simulink subsystem "PMSM_Motor_sref"  (R2025b)
settings: Solver=VariableStepAuto
values from neighbouring files (symbols this model uses):
  B = 1.050e-3    (= 0.00105)    [params_ACT_57BLF02.m]
  J = 1.40e-4    (= 0.00014)    [params_ACT_57BLF02.m]
  Kw = 3.255e-6    (= 3.255e-06)    [params_ACT_57BLF02.m]
  Ld = Ls    (= 0.00019)    [params_ACT_57BLF02.m]
  Lq = Ls    (= 0.00019)    [params_ACT_57BLF02.m]
  p = 4    [params_ACT_57BLF02.m]
  psi = 9.2386e-3    (= 0.0092386)    [params_ACT_57BLF02.m]
  Rs = 0.251    [params_ACT_57BLF02.m]
  T0 = 1.13e-2    (= 0.0113)    [params_ACT_57BLF02.m]
  wth = 1.0    (= 1)    [params_ACT_57BLF02.m]
libraries: simulink x1
settings Model: Creator=Lubin Kerhuel  LastModifiedBy=Lubin Kerhuel

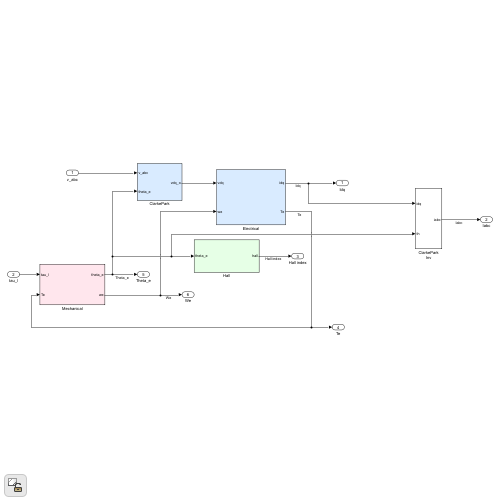
[thumbnail: Simulink's stored preview of the top-level diagram]
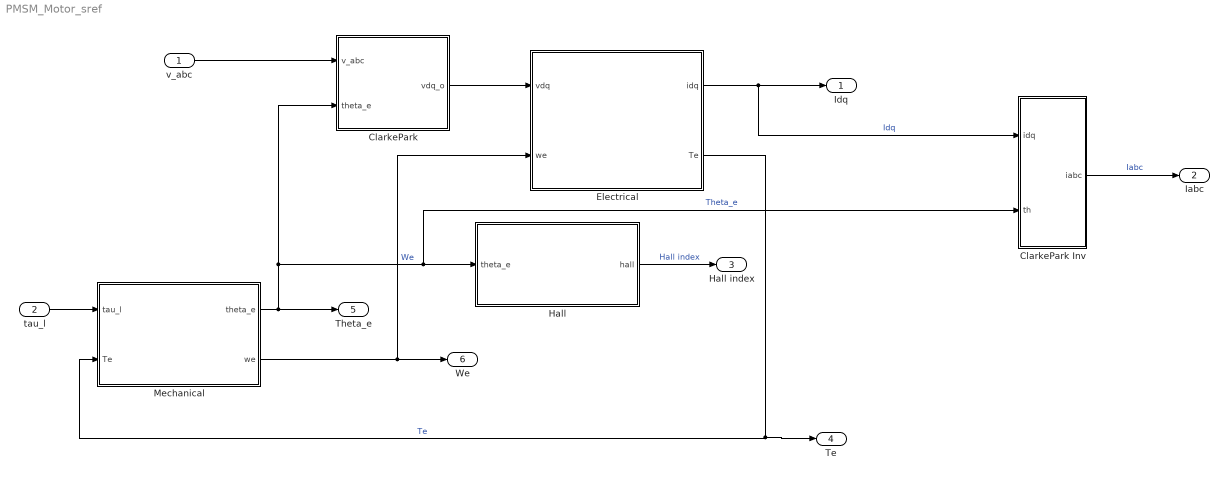
== system PMSM_Motor_sref ==
  v_abc : Inport
  tau_l : Inport  Port=2
  ClarkePark : Subsystem
  ClarkePark Inv : Subsystem
  Electrical : Subsystem
  Hall : Subsystem
  Mechanical : Subsystem
  Idq : Outport
  Iabc : Outport  Port=2
  Hall index : Outport  Port=3
  Te : Outport  Port=4
  Theta_e : Outport  Port=5
  We : Outport  Port=6
  wires:
  ClarkePark/1(vdq_o) -> Electrical/1(vdq)
  ClarkePark Inv/1(iabc) -> Iabc/1  "Iabc"
  tau_l/1 -> Mechanical/1(tau_l)
  v_abc/1 -> ClarkePark/1(v_abc)
  Mechanical/1(theta_e) -> Hall/1(theta_e), ClarkePark Inv/2(th), ClarkePark/2(theta_e), Theta_e/1  "Theta_e"
  Mechanical/2(we) -> Electrical/2(we), We/1  "We"
  Electrical/1(idq) -> ClarkePark Inv/1(idq), Idq/1  "Idq"
  Hall/1(hall) -> Hall index/1  "Hall index"
  Electrical/2(Te) -> Mechanical/2(Te), Te/1  "Te"

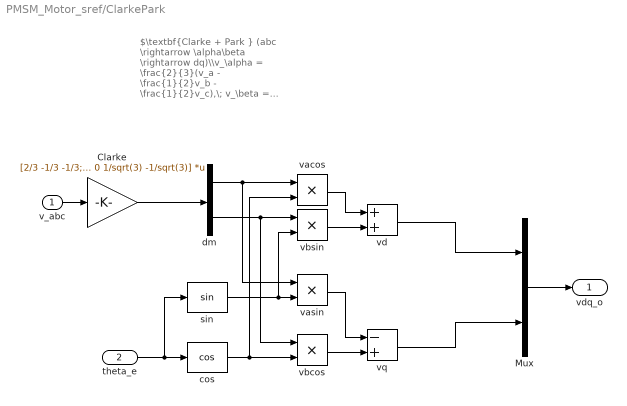
== system PMSM_Motor_sref/ClarkePark ==
  note: $\textbf{Clarke + Park } (abc \rightarrow \alpha\beta \rightarrow dq)\\v_\alpha = \frac{2}{3}(v_a - \frac{1}{2}v_b - \frac{1}{2}v_c),\; v_\beta = \frac{1}{\sqrt{3}}(v_b - v_c)\\v_d = v_\alpha\cos\theta_e + v_\beta\sin\theta_e,\; v_q = -v_\alpha\sin\theta_e + v_\beta\cos\theta_e$
  v_abc : Inport
  theta_e : Inport  Port=2
  Clarke : Gain  Gain=[2/3 -1/3 -1/3; 0 1/sqrt(3) -1/sqrt(3)]  Multiplication=Matrix(K*u)
  Mux : Mux  Inputs=2
  cos : Trigonometry  Operator=cos
  dm : Demux  Outputs=2
  sin : Trigonometry
  vacos : Product  Inputs=**
  vasin : Product  Inputs=**
  vbcos : Product  Inputs=**
  vbsin : Product  Inputs=**
  vd : Sum
  vq : Sum  Inputs=-+
  vdq_o : Outport
  wires:
  Mux/1 -> vdq_o/1
  vd/1 -> Mux/1
  vbcos/1 -> vq/2
  vq/1 -> Mux/2
  vbsin/1 -> vd/2
  dm/1 -> vasin/1, vacos/1
  dm/2 -> vbcos/1, vbsin/1
  cos/1 -> vbcos/2, vacos/2
  vacos/1 -> vd/1
  sin/1 -> vasin/2, vbsin/2
  vasin/1 -> vq/1
  theta_e/1 -> sin/1, cos/1
  v_abc/1 -> Clarke/1
  Clarke/1 -> dm/1

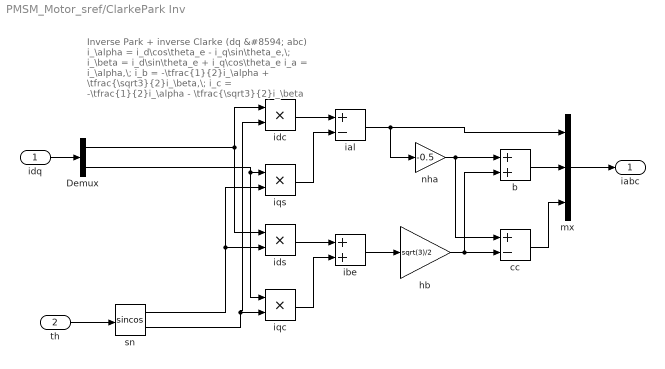
== system PMSM_Motor_sref/ClarkePark Inv ==
  note: Inverse Park + inverse Clarke (dq &#8594; abc)
      | i_\alpha = i_d\cos\theta_e - i_q\sin\theta_e,\; i_\beta = i_d\sin\theta_e + i_q\cos\theta_e
      | i_a = i_\alpha,\; i_b = -\tfrac{1}{2}i_\alpha + \tfrac{\sqrt3}{2}i_\beta,\; i_c = -\tfrac{1}{2}i_\alpha - \tfrac{\sqrt3}{2}i_\beta
  idq : Inport
  th : Inport  Port=2
  Demux : Demux  Outputs=2
  b : Sum
  cc : Sum  Inputs=+-
  hb : Gain  Gain=sqrt(3)/2
  ial : Sum  Inputs=+-
  ibe : Sum
  idc : Product  Inputs=**
  ids : Product  Inputs=**
  iqc : Product  Inputs=**
  iqs : Product  Inputs=**
  mx : Mux  Inputs=3
  nha : Gain  Gain=-0.5
  sn : Trigonometry  Operator=sincos
  iabc : Outport
  wires:
  idq/1 -> Demux/1
  idc/1 -> ial/1
  ids/1 -> ibe/1
  sn/1 -> ids/2, iqs/2
  iqs/1 -> ial/2
  sn/2 -> idc/2, iqc/2
  mx/1 -> iabc/1
  Demux/2 -> iqs/1, iqc/1
  Demux/1 -> idc/1, ids/1
  th/1 -> sn/1
  iqc/1 -> ibe/2
  ial/1 -> mx/1, nha/1
  ibe/1 -> hb/1
  nha/1 -> b/1, cc/1
  cc/1 -> mx/3
  hb/1 -> b/2, cc/2
  b/1 -> mx/2

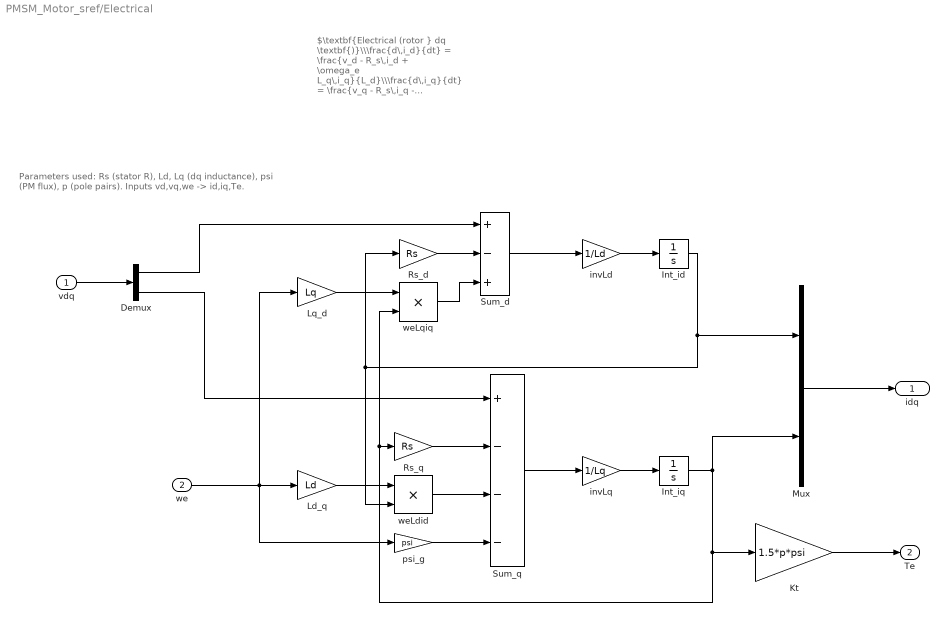
== system PMSM_Motor_sref/Electrical ==
  note: Parameters used: Rs (stator R), Ld, Lq (dq inductance),
      | psi (PM flux), p (pole pairs). Inputs vd,vq,we -> id,iq,Te.
  note: $\textbf{Electrical (rotor } dq \textbf{)}\\\frac{d\,i_d}{dt} = \frac{v_d - R_s\,i_d + \omega_e L_q\,i_q}{L_d}\\\frac{d\,i_q}{dt} = \frac{v_q - R_s\,i_q - \omega_e L_d\,i_d - \omega_e\,\psi}{L_q}\\T_e = \frac{3}{2}\,p\,\psi\,i_q$
  vdq : Inport
  we : Inport  Port=2
  Demux : Demux  Outputs=2
  Int_id : Integrator
  Int_iq : Integrator
  Kt : Gain  Gain=1.5*p*psi
  Ld_q : Gain  Gain=Ld
  Lq_d : Gain  Gain=Lq
  Mux : Mux  Inputs=2
  Rs_d : Gain  Gain=Rs
  Rs_q : Gain  Gain=Rs
  Sum_d : Sum  Inputs=+-+
  Sum_q : Sum  Inputs=+---
  invLd : Gain  Gain=1/Ld
  invLq : Gain  Gain=1/Lq
  psi_g : Gain  Gain=psi
  weLdid : Product
  weLqiq : Product
  idq : Outport
  Te : Outport  Port=2
  wires:
  Mux/1 -> idq/1
  Demux/1 -> Sum_d/1
  vdq/1 -> Demux/1
  Kt/1 -> Te/1
  Ld_q/1 -> weLdid/1
  invLq/1 -> Int_iq/1
  Sum_q/1 -> invLq/1
  psi_g/1 -> Sum_q/4
  weLdid/1 -> Sum_q/3
  Rs_q/1 -> Sum_q/2
  Demux/2 -> Sum_q/1
  Int_iq/1 -> Mux/2, Rs_q/1, weLqiq/2, Kt/1
  Lq_d/1 -> weLqiq/1
  we/1 -> Ld_q/1, psi_g/1, Lq_d/1
  Int_id/1 -> Mux/1, Rs_d/1, weLdid/2
  invLd/1 -> Int_id/1
  Sum_d/1 -> invLd/1
  weLqiq/1 -> Sum_d/3
  Rs_d/1 -> Sum_d/2

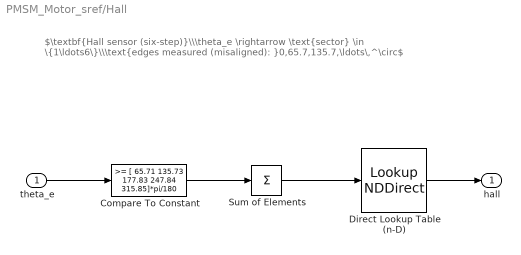
== system PMSM_Motor_sref/Hall ==
  note: $\textbf{Hall sensor (six-step)}\\\theta_e \rightarrow \text{sector} \in \{1\ldots6\}\\\text{edges measured (misaligned): }0,65.7,135.7,\ldots\,^\circ$
  theta_e : Inport
  Compare To Constant : simulink/Logic and Bit Operations/Compare To Constant  relop=>=  const="[  65.71 135.73 177.83 247.84 315.85]*pi/180"  OutDataTypeStr=boolean
  Direct Lookup Table (n-D) : LookupNDDirect  NumberOfTableDimensions=1  Table=[ 4 6 2 3 1 5 ];
  Sum of Elements : Sum  Inputs=+
  hall : Outport
  wires:
  Direct Lookup Table (n-D)/1 -> hall/1
  Sum of Elements/1 -> Direct Lookup Table (n-D)/1
  Compare To Constant/1 -> Sum of Elements/1
  theta_e/1 -> Compare To Constant/1

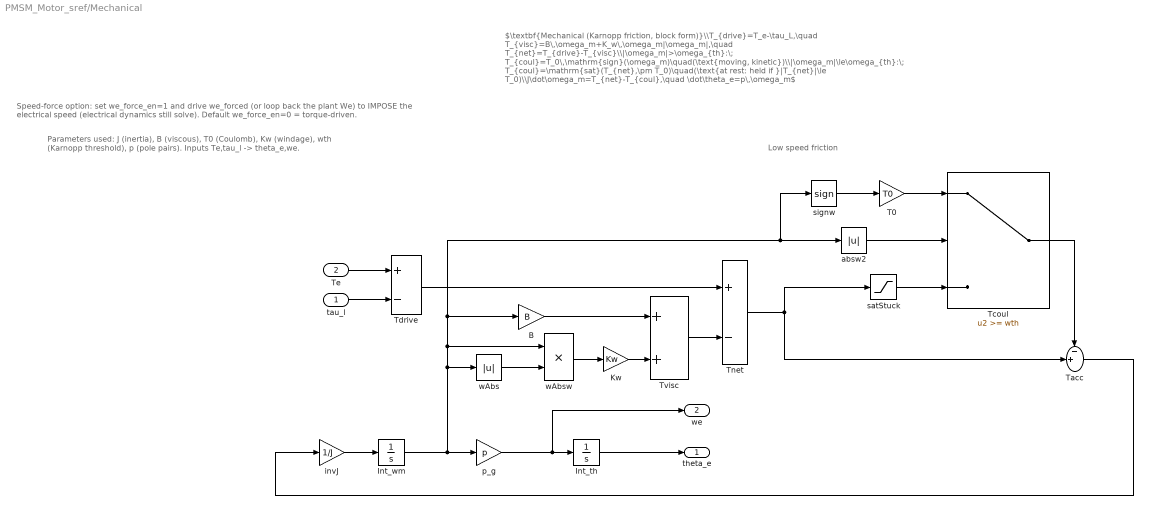
== system PMSM_Motor_sref/Mechanical ==
  note: Speed-force option: set we_force_en=1 and drive we_forced (or loop back the plant We)
      | to IMPOSE the electrical speed (electrical dynamics still solve). Default we_force_en=0 = torque-driven.
  note: Parameters used: J (inertia), B (viscous),
      | T0 (Coulomb), Kw (windage), wth (Karnopp threshold), p (pole pairs).
      | Inputs Te,tau_l -> theta_e,we.
  note: $\textbf{Mechanical (Karnopp friction, block form)}\\T_{drive}=T_e-\tau_L,\quad T_{visc}=B\,\omega_m+K_w\,\omega_m|\omega_m|,\quad T_{net}=T_{drive}-T_{visc}\\|\omega_m|>\omega_{th}:\; T_{coul}=T_0\,\mathrm{sign}(\omega_m)\quad(\text{moving, kinetic})\\|\omega_m|\le\omega_{th}:\; T_{coul}=\mathrm{sat}(T_{net},\pm T_0)\quad(\text{at rest: held if }|T_{net}|\le T_0)\\J\dot\omega_m=T_{net}-T_{coul},\quad \dot\theta_e=p\,\omega_m$
  note: Low speed friction
  tau_l : Inport
  Te : Inport  Port=2
  B : Gain  Gain=B
  Int_th : Integrator  WrapState=on  WrappedStateUpperValue=2*pi  WrappedStateLowerValue=0
  Int_wm : Integrator
  Kw : Gain  Gain=Kw
  T0 : Gain  Gain=T0
  Tacc : Sum  Inputs=-+|
  Tcoul : Switch  Threshold=wth  SaturateOnIntegerOverflow=off  InputSameDT=off
  Tdrive : Sum  Inputs=+-
  Tnet : Sum  Inputs=+-
  Tvisc : Sum
  absw2 : Abs  SaturateOnIntegerOverflow=off
  invJ : Gain  Gain=1/J
  p_g : Gain  Gain=p
  satStuck : Saturate  UpperLimit=T0  LowerLimit=-T0
  signw : Signum
  wAbs : Abs  SaturateOnIntegerOverflow=off
  wAbsw : Product  Inputs=**
  theta_e : Outport
  we : Outport  Port=2
  wires:
  Tacc/1 -> invJ/1
  Tcoul/1 -> Tacc/1
  satStuck/1 -> Tcoul/3
  absw2/1 -> Tcoul/2
  T0/1 -> Tcoul/1
  Tnet/1 -> satStuck/1, Tacc/2
  Tvisc/1 -> Tnet/2
  Tdrive/1 -> Tnet/1
  Kw/1 -> Tvisc/2
  B/1 -> Tvisc/1
  wAbsw/1 -> Kw/1
  wAbs/1 -> wAbsw/2
  tau_l/1 -> Tdrive/2
  Te/1 -> Tdrive/1
  Int_th/1 -> theta_e/1
  invJ/1 -> Int_wm/1
  p_g/1 -> Int_th/1, we/1
  Int_wm/1 -> p_g/1, wAbs/1, wAbsw/1, B/1, absw2/1, signw/1
  signw/1 -> T0/1
